simulink model "Load_Flow_Analysis"  (R2023b)
settings: Solver=ode45  StartTime=0.0  StopTime=1  MaxStep=1e-4  RelTol=1e-3
undefined symbols (not defined in the file or in its folder): Angle, Magnitude
libraries: spsThreePhaseVIMeasurementLib x3, spsLoadFlowBusLib x3, spsThreePhaseSeriesRLCBranchLib x3, spsThreePhaseParallelRLCLoadLib x2, spsThreePhaseSourceLib x1, spspowerguiLib x1
settings Model: Creator=HP  LastModifiedBy=HP
settings SolverCC: AlgebraicLoopSolver=TrustRegion
settings DataIOCC: ReturnWorkspaceOutputs=off
settings DebuggingCC: UnconnectedInputMsg=warning  UnconnectedOutputMsg=warning  UnconnectedLineMsg=warning  ArithmeticOperatorsInVariantConditions=warning
settings ModelReferenceCC: EnableRefExpFcnMdlSchedulingChecks=on
settings SFSimCC: SimUseLocalCustomCode=off  CustomCodeUndefinedFunction=UseInterfaceOnly
settings RTWCC: RTWUseLocalCustomCode=off
settings CodeAppCC: StateflowObjectComments=on
settings SimscapeCC: SimscapeNormalizeSystem=off

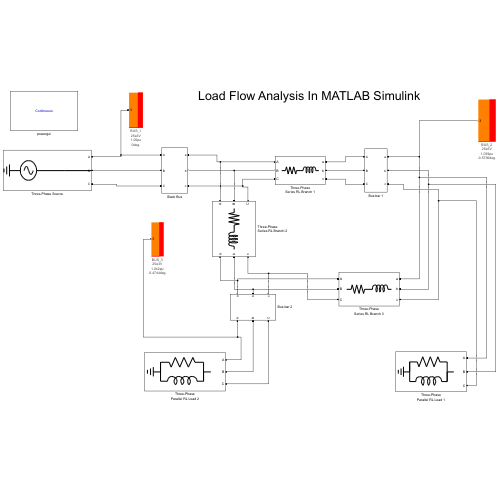
[thumbnail: Simulink's stored preview of the top-level diagram]
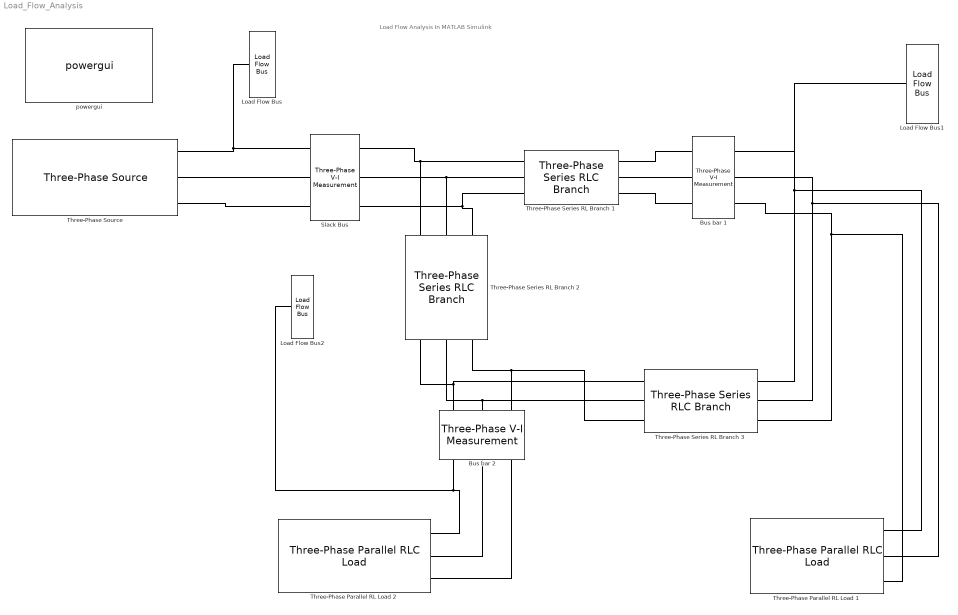
== system Load_Flow_Analysis ==
  note: Load Flow Analysis In MATLAB Simulink
  Bus bar 1 : spsThreePhaseVIMeasurementLib/Three-Phase V-I Measurement  VoltageMeasurement=no  SetLabelV=off  LabelV=Vabc  Vpu=off  VpuLL=on  CurrentMeasurement=no  SetLabelI=off  LabelI=Iabc  Ipu=on  Pbase=100e6  Vbase=25e3  OutputType=Magnitude  PhasorSimulation=off  PSBequivalent=0
  Bus bar 2 : spsThreePhaseVIMeasurementLib/Three-Phase V-I Measurement  VoltageMeasurement=no  SetLabelV=off  LabelV=Vabc  Vpu=off  VpuLL=on  CurrentMeasurement=no  SetLabelI=off  LabelI=Iabc  Ipu=off  Pbase=100e6  Vbase=11e3  OutputType=Magnitude-Angle  PhasorSimulation=off  PSBequivalent=0
  Load Flow Bus : spsLoadFlowBusLib/Load Flow Bus  LConnTagsString=a  Phases=single  Connectors=on one side  ID=BUS_1  Vbase=25e3  Vref=1.05  Vangle=0  VLF=1.05  VLFb=1  VLFc=1  angleLF=0  angleLFb=0  angleLFc=0
  Load Flow Bus1 : spsLoadFlowBusLib/Load Flow Bus  LConnTagsString=a  Phases=single  Connectors=on one side  ID=BUS_2  Vbase=25e3  Vref=1  Vangle=0  VLF=1.039  VLFb=1  VLFc=1  angleLF=-0.5736  angleLFb=0  angleLFc=0
  Load Flow Bus2 : spsLoadFlowBusLib/Load Flow Bus  LConnTagsString=a  Phases=single  Connectors=on one side  ID=BUS_3  Vbase=25e3  Vref=1  Vangle=0  VLF=1.042  VLFb=1  VLFc=1  angleLF=-0.4744  angleLFb=0  angleLFc=0
  Slack Bus : spsThreePhaseVIMeasurementLib/Three-Phase V-I Measurement  VoltageMeasurement=no  SetLabelV=off  LabelV=Vabc  Vpu=off  VpuLL=on  CurrentMeasurement=no  SetLabelI=off  LabelI=Iabc  Ipu=on  Pbase=100e6  Vbase=25e3  OutputType=Magnitude-Angle  PhasorSimulation=off  PSBequivalent=0
  Three-Phase Parallel RL Load 1 : spsThreePhaseParallelRLCLoadLib/Three-Phase Parallel RLC Load  LConnTagsString=A|B|C  Configuration=Y (grounded)  NominalVoltage=25e3  Vabc=[1e3 1e3 1e3]  Vabcp=[1e3 1e3 1e3]  NominalFrequency=60  UnbalancedPower=off  ActivePower=256.6e6  InductivePower=110.2e6  CapacitivePower=0  Pabc=[10e3 9e3 11e3]  QLabc=[100 90 110]  QCabc=[100 90 110]  Pabcp=[10e3 9e3 11e3]  QLabcp=[100 90 110]  QCabcp=[100 90 110]  Measurements=None  LoadType=constant PQ
  Three-Phase Parallel RL Load 2 : spsThreePhaseParallelRLCLoadLib/Three-Phase Parallel RLC Load  LConnTagsString=A|B|C  Configuration=Y (grounded)  NominalVoltage=25e3  Vabc=[1e3 1e3 1e3]  Vabcp=[1e3 1e3 1e3]  NominalFrequency=60  UnbalancedPower=off  ActivePower=138.6e6  InductivePower=45.2e6  CapacitivePower=0  Pabc=[10e3 9e3 11e3]  QLabc=[100 90 110]  QCabc=[100 90 110]  Pabcp=[10e3 9e3 11e3]  QLabcp=[100 90 110]  QCabcp=[100 90 110]  Measurements=None  LoadType=constant PQ
  Three-Phase Series RL Branch 1 : spsThreePhaseSeriesRLCBranchLib/Three-Phase Series RLC Branch  LConnTagsString=A|B|C  RConnTagsString=A|B|C  BranchType=RL  Resistance=0.02*6.25  Inductance=(0.04*6.25)/(2*pi*60)  Capacitance=1e-6  Measurements=Branch voltages and currents
  Three-Phase Series RL Branch 2 : spsThreePhaseSeriesRLCBranchLib/Three-Phase Series RLC Branch  LConnTagsString=A|B|C  RConnTagsString=A|B|C  BranchType=RL  Resistance=0.01*6.25  Inductance=(0.03*6.25)/(2*pi*60)  Capacitance=1e-6  Measurements=Branch voltages and currents
  Three-Phase Series RL Branch 3 : spsThreePhaseSeriesRLCBranchLib/Three-Phase Series RLC Branch  LConnTagsString=A|B|C  RConnTagsString=A|B|C  BranchType=RL  Resistance=0.0125*6.25  Inductance=(0.025*6.25)/(2*pi*60)  Capacitance=1e-6  Measurements=Branch voltages and currents
  Three-Phase Source : spsThreePhaseSourceLib/Three-Phase Source  InternalConnection=Yg  VoltagePhases=off  Voltage=1.05*25000  PhaseAngle=0  Voltage_phases=[25e3 25e3 25e3]/sqrt(3)  PhaseAngles_phases=[0 -120 +120]  Frequency=60  NonIdealSource=off  SpecifyImpedance=off  Resistance=0.8929  Inductance=16.58e-3  ShortCircuitLevel=100e6  BaseVoltage=25e3  XRratio=7  BusType=swing  Pref=10e3  Qref=0  Prefabc=[10e3, 10e3, 10e3]  Qrefabc=[0, 0, 0]  Qmin=-inf  Qmax=inf
  powergui : spspowerguiLib/powergui  Priority=1  SimulationMode=Continuous  SampleTime=50e-6  frequency=60  Iterations=50  frequencyindice=60  Pbase=100e6  ErrMax=0.0001  UnitsV=kV  UnitsW=MW  buscounter=0  FunctionMessages=off  echomessages=off  EnableUseOfTLC=off  CurrentSourceSwitches=off  DisableSnubberDevices=off  DisableRonSwitches=off  DisableVfSwitches=off  DisplayEquations=off  AutomaticDiscreteSolvers=off  SolverType=Tustin/Backward Euler (TBE)  Interpol=off  ExternalGateDelay=off  methode=off  Ts=100  x0status=blocks  SPID=on  SwTol=0  HookPort=off  NonlinearTolerance=1e-4  nMaxIteration=100  ContinueOnMaxIteration=off  RestoreLinks=warning  ResistiveCurrentMeasurement=off  Frange=[0:2:500]  Ylog=off  Xlog=on  ShowGrid=off  save=off  variable=ZData  structure=0  ZoomFFT=off  StartTime=0.0  cycles=1  DisplayStyle=1  fundamental=60  FreqAxis=off  MaxFrequency=1000  frequencyindicesteady=1  RmsSteady=1  display=off
  connections:
  Slack Bus/LConn1 -- Load Flow Bus/LConn1 -- Three-Phase Source/RConn1
  Three-Phase Source/RConn2 -- Slack Bus/LConn2
  Three-Phase Source/RConn3 -- Slack Bus/LConn3
  Three-Phase Series RL Branch 1/LConn1 -- Slack Bus/RConn1 -- Three-Phase Series RL Branch 2/LConn1
  Three-Phase Series RL Branch 2/LConn2 -- Slack Bus/RConn2 -- Three-Phase Series RL Branch 1/LConn2
  Three-Phase Series RL Branch 1/LConn3 -- Three-Phase Series RL Branch 2/LConn3 -- Slack Bus/RConn3
  Three-Phase Series RL Branch 3/RConn2 -- Bus bar 1/RConn2 -- Three-Phase Parallel RL Load 1/LConn2
  Three-Phase Series RL Branch 3/RConn1 -- Load Flow Bus1/LConn1 -- Bus bar 1/RConn1 -- Three-Phase Parallel RL Load 1/LConn1
  Three-Phase Series RL Branch 3/RConn3 -- Bus bar 1/RConn3 -- Three-Phase Parallel RL Load 1/LConn3
  Bus bar 2/RConn1 -- Three-Phase Series RL Branch 3/LConn1 -- Three-Phase Series RL Branch 2/RConn1
  Bus bar 2/RConn2 -- Three-Phase Series RL Branch 2/RConn2 -- Three-Phase Series RL Branch 3/LConn2
  Bus bar 2/RConn3 -- Three-Phase Series RL Branch 2/RConn3 -- Three-Phase Series RL Branch 3/LConn3
  Load Flow Bus2/LConn1 -- Three-Phase Parallel RL Load 2/LConn1 -- Bus bar 2/LConn1
  Three-Phase Parallel RL Load 2/LConn2 -- Bus bar 2/LConn2
  Three-Phase Parallel RL Load 2/LConn3 -- Bus bar 2/LConn3
  Bus bar 1/LConn1 -- Three-Phase Series RL Branch 1/RConn1
  Three-Phase Series RL Branch 1/RConn2 -- Bus bar 1/LConn2
  Three-Phase Series RL Branch 1/RConn3 -- Bus bar 1/LConn3
